simulink model "SignosPatologia"  (R2020a)
settings: Solver=FixedStepAuto  StartTime=0.0  StopTime=10.0  RelTol=1e-3
undefined symbols (not defined in the file): A1, alphaCo2, c1, c2, c3, Ca, Ce, Ci, Cv, d, Ed, epsilon, Es0, gananciaOut, K, offsetMaxFinder, omega0, Pex, picoR, Pset, Ra, Re0, Ri, Rlv, Rv, T, tau, tau1, tau2, Tdia, Ve0
libraries: androiduilib x6, simulink x4, dspswit3 x2
settings Model: Creator=luisi  LastModifiedBy=luisi
settings OptimizationCC: EnhancedBackFolding=on  PassReuseOutputArgsAs=Individual arguments  ZeroExternalMemoryAtStartup=off  ZeroInternalMemoryAtStartup=off  MaxStackSize=64  OptimizeBlockOrder=speed  DifferentSizesBufferReuse=on  OptimizationCustomize=off  EfficientTunableParamExpr=on
settings DebuggingCC: ParameterTunabilityLossMsg=error
settings HardwareCC: ProdBitPerPointer=32  ProdBitPerSizeT=32  ProdBitPerPtrDiffT=32  ProdLargestAtomicInteger=Long  ProdLargestAtomicFloat=Double  ProdWordSize=32  ProdHWDeviceType=ARM Compatible->ARM Cortex
settings SFSimCC: MATLABDynamicMemAlloc=off
settings RTWCC: SystemTargetFile=ert.tlc  HardwareBoard=Android Device  TemplateMakefile=ert_default_tmf  RTWVerbose=off  Toolchain=Android SDK/NDK Tools
settings CodeAppCC: ForceParamTrailComments=on  IgnoreCustomStorageClasses=off  OperatorAnnotations=on  SimulinkDataObjDesc=on  SFDataObjDesc=on  InsertBlockDesc=on
settings ERTTargetCC: SupportContinuousTime=on

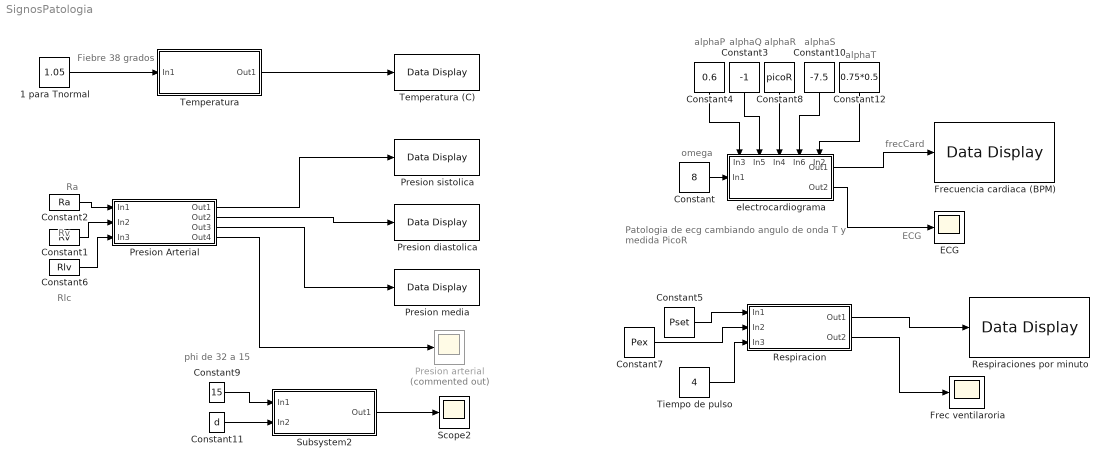
== system SignosPatologia ==
  note: Ra
  note: phi de 32 a 15
  note: Patologia de ecg cambiando angulo de onda T
      |  y medida PicoR
  note: Fiebre 38 grados
  note: alphaR
  note: ECG
  note: alphaQ
  note: alphaP
  note: alphaT
  note: alphaS
  note: omega
  note: frecCard
  note: Rv
  note: Rlc
  1 para Tnormal : Constant  Value=1.05
  Constant : Constant  Value=8
  Constant1 : Constant  Value=Rv
  Constant10 : Constant  Value=-7.5
  Constant11 : Constant  Value=d
  Constant12 : Constant  Value=0.75*0.5
  Constant2 : Constant  Value=Ra
  Constant3 : Constant  Value=-1
  Constant4 : Constant  Value=0.6
  Constant5 : Constant  Value=Pset
  Constant6 : Constant  Value=Rlv
  Constant7 : Constant  Value=Pex
  Constant8 : Constant  Value=picoR
  Constant9 : Constant  Value=15
  ECG : Scope
      settings: AttributesFormatString=%<AxesScaling>
  Frec ventilaroria : Scope
  Frecuencia cardiaca (BPM) : androiduilib/Data Display  DataDisplayId=SignosPatologia/Frecuencia_cardiaca_(BPM)  Format=Float  Precision=6  SimulateUsing=Code generation  blockPlatform=Android
      settings: SourceProductBaseCode=ANDROID
  Presion Arterial : Subsystem
  Presion arterial : Scope  Commented=on
  Presion diastolica : androiduilib/Data Display  DataDisplayId=SignosPatologia/Presion_diastolica  Format=Float  Precision=6  SimulateUsing=Code generation  blockPlatform=Android
      settings: SourceProductBaseCode=ANDROID
  Presion media : androiduilib/Data Display  DataDisplayId=SignosPatologia/Presion_media  Format=Float  Precision=6  SimulateUsing=Code generation  blockPlatform=Android
      settings: SourceProductBaseCode=ANDROID
  Presion sistolica : androiduilib/Data Display  DataDisplayId=SignosPatologia/Presion_sistolica  Format=Float  Precision=6  SimulateUsing=Code generation  blockPlatform=Android
      settings: SourceProductBaseCode=ANDROID
  Respiracion : Subsystem
  Respiraciones por minuto : androiduilib/Data Display  DataDisplayId=SignosPatologia/Respiraciones_por_minuto  Format=Float  Precision=6  SimulateUsing=Code generation  blockPlatform=Android
      settings: SourceProductBaseCode=ANDROID
  Scope2 : Scope
  Subsystem2 : Subsystem
  Temperatura : Subsystem
  Temperatura (C) : androiduilib/Data Display  DataDisplayId=SignosPatologia/Temperatura_(C)  Format=Float  Precision=6  SimulateUsing=Code generation  blockPlatform=Android
      settings: SourceProductBaseCode=ANDROID
  Tiempo de pulso : Constant  Value=4
  electrocardiograma : Subsystem
      settings: PortSchema="{\"entries\":[{\"content\":{\"sides\":[{\"content\":{\"connectorIds\":[\"In1\"]},\"type\":\"ConnectorPlacement.EquallySpacedRectSide\",\"uuid\":\"28011a65-da2e-41a8-8a5a-207c074f97f9\"},{\"content\":{\"connectorIds\":[\"Out1\",\"Out2\"],\"side\":\"RIGHT\"},\"type\":\"ConnectorPlacement.EquallySpacedRectSide\",\"uuid\":\"adec610a-f47f-48bc-af05-027a0272bce0\"},{\"content\":{\"connectorIds\":[\"In2\",\"In3\",\"In4\",\"In5\",\"In6\"],\"side\":\"TOP\"},\"type\":\"ConnectorPlacement.EquallySpacedRectSide\",\"uuid\":\"45565275-fa9c-45e2-aeb7-03b042b7619a\"}]},\"type\":\"ConnectorPlacement.EquallySpacedConnector\",\"uuid\":\"6408496b-6851-4df8-8646-e1f498398f76\"}],\"packageUris\":[\"http://schema.mathworks.com/mf0/Connector/19700101\"],\"version\":\"1.0\"}"
  wires:
  Temperatura/1(Out1) -> Temperatura (C)/1
  1 para Tnormal/1 -> Temperatura/1(In1)
  Presion Arterial/2(Out2) -> Presion diastolica/1
  Presion Arterial/3(Out3) -> Presion media/1
  Constant2/1 -> Presion Arterial/1(In1)
  Constant6/1 -> Presion Arterial/3(In3)
  Presion Arterial/1(Out1) -> Presion sistolica/1
  Constant1/1 -> Presion Arterial/2(In2)
  Constant8/1 -> electrocardiograma/4(In4)
  Constant/1 -> electrocardiograma/1(In1)
  electrocardiograma/1(Out1) -> Frecuencia cardiaca (BPM)/1
  electrocardiograma/2(Out2) -> ECG/1
  Constant4/1 -> electrocardiograma/2(In3)
  Constant12/1 -> electrocardiograma/6(In2)
  Constant10/1 -> electrocardiograma/5(In6)
  Constant3/1 -> electrocardiograma/3(In5)
  Presion Arterial/4(Out4) -> Presion arterial/1
  Constant7/1 -> Respiracion/2(In2)
  Constant5/1 -> Respiracion/1(In1)
  Respiracion/1(Out1) -> Respiraciones por minuto/1
  Respiracion/2(Out2) -> Frec ventilaroria/1
  Tiempo de pulso/1 -> Respiracion/3(In3)
  Constant9/1 -> Subsystem2/1(In1)
  Subsystem2/1(Out1) -> Scope2/1
  Constant11/1 -> Subsystem2/2(In2)

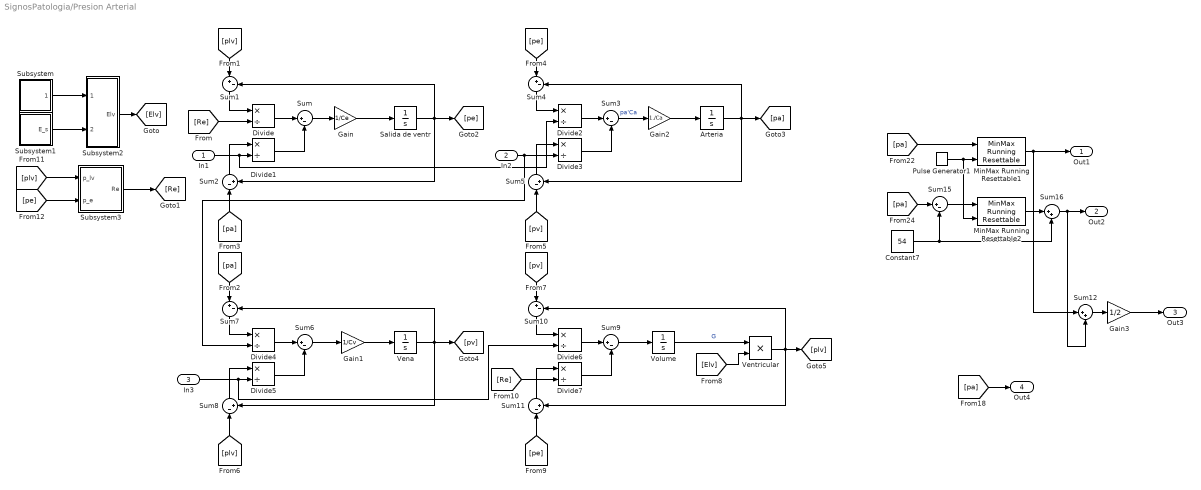
== system SignosPatologia/Presion Arterial ==
  In1 : Inport
  In2 : Inport  Port=2
  In3 : Inport  Port=3
  Arteria : Integrator  InitialCondition=70
  Constant7 : Constant  Value=54
  Divide{,1..7} (8 alike) : Product  Inputs=*/
  Gain : Gain  Gain=1/Ce
  Gain1 : Gain  Gain=1/Cv
  Gain2 : Gain  Gain=1./Ca
  Gain3 : Gain  Gain=1/2
  MinMax Running Resettable1 : simulink/Math Operations/MinMax Running Resettable  Function=max  vinit=70
  MinMax Running Resettable2 : simulink/Math Operations/MinMax Running Resettable  Function=min  vinit=0.0
  Pulse Generator1 : DiscretePulseGenerator  PulseType=Time based  Period=8  PulseWidth=5
  Salida de ventr : Integrator  InitialCondition=49.896
  Subsystem : Subsystem
  Subsystem1 : Subsystem
  Subsystem2 : Subsystem
  Subsystem3 : Subsystem
  Sum{,1,3..4,6..7,9..10,15} (9 alike) : Sum  Inputs=|+-
  Sum{2,5,8,11} (4 alike) : Sum  Inputs=|-+
  Sum12 : Sum  Inputs=|++
  Sum16 : Sum  Inputs=|++
  Vena : Integrator  InitialCondition=16.628
  Ventricular : Product
  Volume : Integrator  InitialCondition=49.714/0.0655
  Out1 : Outport
  Out2 : Outport  Port=2
  Out3 : Outport  Port=3
  Out4 : Outport  Port=4
  wires:
  Sum12/1 -> Gain3/1
  Gain3/1 -> Out3/1
  Sum16/1 -> Sum12/2, Out2/1
  MinMax Running Resettable2/1 -> Sum16/1
  Sum3/1 -> Gain2/1  "pa'Ca"
  [pa] -> MinMax Running Resettable1/1
  Sum10/1 -> Divide6/1
  MinMax Running Resettable1/1 -> Sum12/1, Out1/1
  Subsystem2/1(Elv) -> [Elv]
  Constant7/1 -> Sum16/2, Sum15/2
  Salida de ventr/1 -> [pe], Sum2/2, Sum1/2
  [pa] -> Sum15/1
  Divide6/1 -> Sum9/1
  Pulse Generator1/1 -> MinMax Running Resettable2/2, MinMax Running Resettable1/2
  [Elv] -> Ventricular/2
  [pa] -> Out4/1
  Gain/1 -> Salida de ventr/1
  [Re] -> Divide/2
  In2/1 -> Divide4/2, Divide3/2
  Sum5/1 -> Divide3/1
  [plv] -> Subsystem3/1(p_lv)
  Divide/1 -> Sum/1
  [plv] -> Sum1/1
  [pv] -> Sum10/1
  Ventricular/1 -> Sum10/2, [plv], Sum11/2
  Sum15/1 -> MinMax Running Resettable2/1
  [pe] -> Sum4/1
  [pe] -> Subsystem3/2(p_e)
  Sum9/1 -> Volume/1
  [plv] -> Sum8/1
  Gain1/1 -> Vena/1
  [pv] -> Sum5/1
  Divide7/1 -> Sum9/2
  In3/1 -> Divide6/2, Divide5/2
  Gain2/1 -> Arteria/1
  Sum8/1 -> Divide5/1
  Sum11/1 -> Divide7/1
  Divide2/1 -> Sum3/1
  [pe] -> Sum11/1
  [pa] -> Sum7/1
  Sum7/1 -> Divide4/1
  Vena/1 -> [pv], Sum8/2, Sum7/2
  Divide3/1 -> Sum3/2
  Sum6/1 -> Gain1/1
  Volume/1 -> Ventricular/1  "G"
  Divide5/1 -> Sum6/2
  Divide4/1 -> Sum6/1
  Arteria/1 -> Sum5/2, Sum4/2, [pa]
  [pa] -> Sum2/1
  [Re] -> Divide7/2
  Sum2/1 -> Divide1/1
  Sum1/1 -> Divide/1
  Sum/1 -> Gain/1
  Sum4/1 -> Divide2/1
  Subsystem3/1(Re) -> [Re]
  Subsystem/1(alpha_t) -> Subsystem2/1(alpha)
  Subsystem1/1(E_s) -> Subsystem2/2(E_s)
  Divide1/1 -> Sum/2
  In1/1 -> Divide2/2, Divide1/2

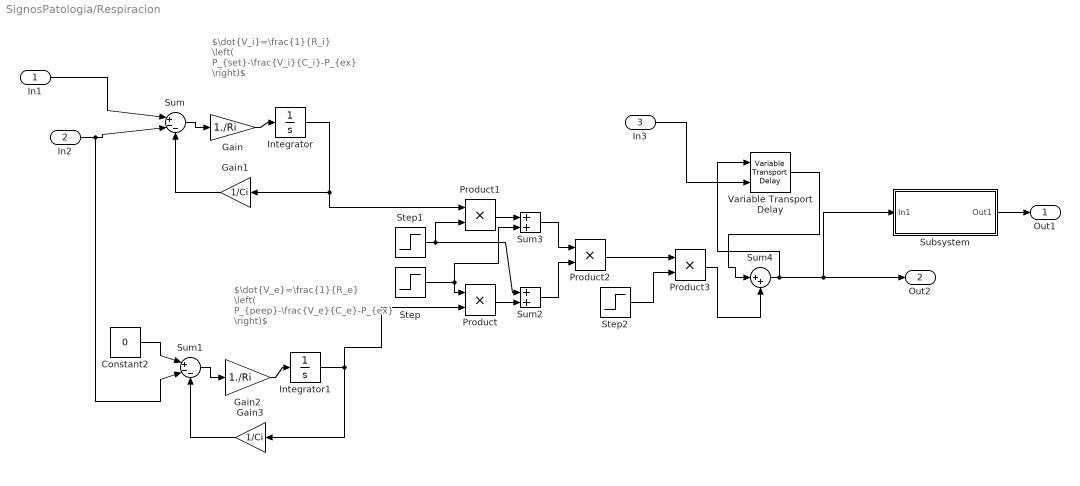
== system SignosPatologia/Respiracion ==
  note: $\dot{V_i}=\frac{1}{R_i} \left( P_{set}-\frac{V_i}{C_i}-P_{ex} \right)$
  note: $\dot{V_e}=\frac{1}{R_e} \left( P_{peep}-\frac{V_e}{C_e}-P_{ex} \right)$
  In1 : Inport
  In2 : Inport  Port=2
  In3 : Inport  Port=3
  Constant2 : Constant  Value=0
  Gain : Gain  Gain=1./Ri
  Gain1 : Gain  Gain=1/Ci
  Gain2 : Gain  Gain=1./Ri
  Gain3 : Gain  Gain=1/Ci
  Integrator : Integrator
  Integrator1 : Integrator  InitialCondition=Ve0
  Product{,1..3} (4 alike) : Product
  Step : Step  Time=2  SampleTime=0
  Step1 : Step  Time=2  Before=1  After=0  SampleTime=0
  Step2 : Step  Time=4  Before=1  After=0  SampleTime=0
  Subsystem : Subsystem
  Sum : Sum  Inputs=|+--
  Sum1 : Sum  Inputs=|+--
  Sum2 : Sum
  Sum3 : Sum
  Sum4 : Sum  Inputs=|++
  Variable Transport Delay : VariableTransportDelay  VariableDelayType=Variable transport delay  MaximumDelay=10
  Out1 : Outport
  Out2 : Outport  Port=2
  wires:
  Sum3/1 -> Product2/1
  Sum2/1 -> Product2/2
  Gain3/1 -> Sum1/3
  Integrator1/1 -> Product/2, Gain3/1
  Product2/1 -> Product3/1
  Product1/1 -> Sum3/1
  Step2/1 -> Product3/2
  Product3/1 -> Sum4/2
  Integrator/1 -> Product1/1, Gain1/1
  Step/1 -> Product/1, Sum3/2
  Product/1 -> Sum2/2
  Sum4/1 -> Variable Transport Delay/1, Out2/1, Subsystem/1(In1)
  Gain2/1 -> Integrator1/1
  Variable Transport Delay/1 -> Sum4/1
  Gain1/1 -> Sum/3
  Subsystem/1(Out1) -> Out1/1
  Sum1/1 -> Gain2/1
  Step1/1 -> Sum2/1, Product1/2
  In2/1 -> Sum1/2, Sum/2
  Constant2/1 -> Sum1/1
  Gain/1 -> Integrator/1
  Sum/1 -> Gain/1
  In1/1 -> Sum/1
  In3/1 -> Variable Transport Delay/2

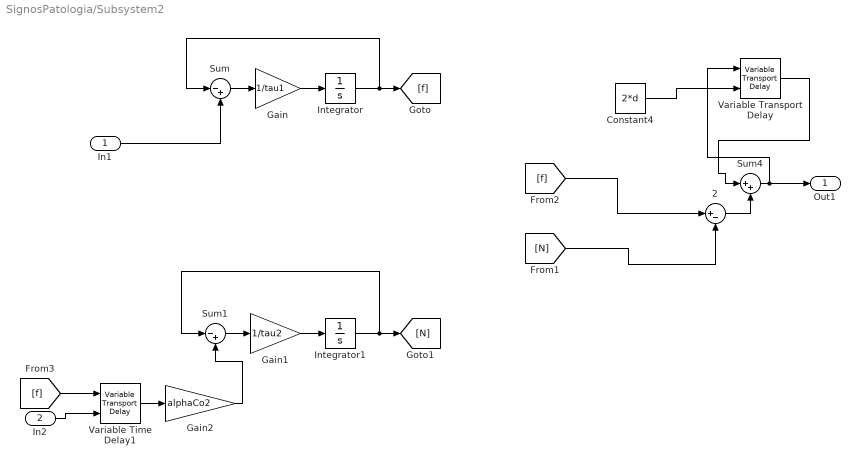
== system SignosPatologia/Subsystem2 ==
  In1 : Inport
  In2 : Inport  Port=2
  2 : Sum  Inputs=|+-
  Constant4 : Constant  Value=2*d
  Gain : Gain  Gain=1/tau1
  Gain1 : Gain  Gain=1/tau2
  Gain2 : Gain  Gain=alphaCo2
  Integrator : Integrator
  Integrator1 : Integrator
  Sum : Sum  Inputs=|-+
  Sum1 : Sum  Inputs=|-+
  Sum4 : Sum  Inputs=|++
  Variable Time Delay1 : VariableTransportDelay  MaximumDelay=10
  Variable Transport Delay : VariableTransportDelay  VariableDelayType=Variable transport delay  MaximumDelay=10
  Out1 : Outport
  wires:
  In1/1 -> Sum/2
  Sum1/1 -> Gain1/1
  Gain1/1 -> Integrator1/1
  Integrator1/1 -> [N], Sum1/1
  Sum4/1 -> Out1/1, Variable Transport Delay/1
  Integrator/1 -> [f], Sum/1
  Gain/1 -> Integrator/1
  Constant4/1 -> Variable Transport Delay/2
  [f] -> 2/1
  [N] -> 2/2
  [f] -> Variable Time Delay1/1
  Gain2/1 -> Sum1/2
  Sum/1 -> Gain/1
  Variable Transport Delay/1 -> Sum4/1
  In2/1 -> Variable Time Delay1/2
  2/1 -> Sum4/2
  Variable Time Delay1/1 -> Gain2/1

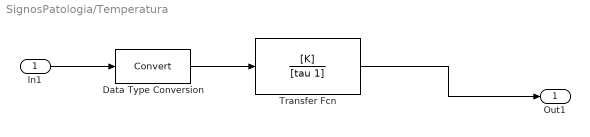
== system SignosPatologia/Temperatura ==
  In1 : Inport
  Data Type Conversion : DataTypeConversion
  Transfer Fcn : TransferFcn  Numerator=[K]  Denominator=[tau 1]
  Out1 : Outport
  wires:
  Data Type Conversion/1 -> Transfer Fcn/1
  Transfer Fcn/1 -> Out1/1
  In1/1 -> Data Type Conversion/1

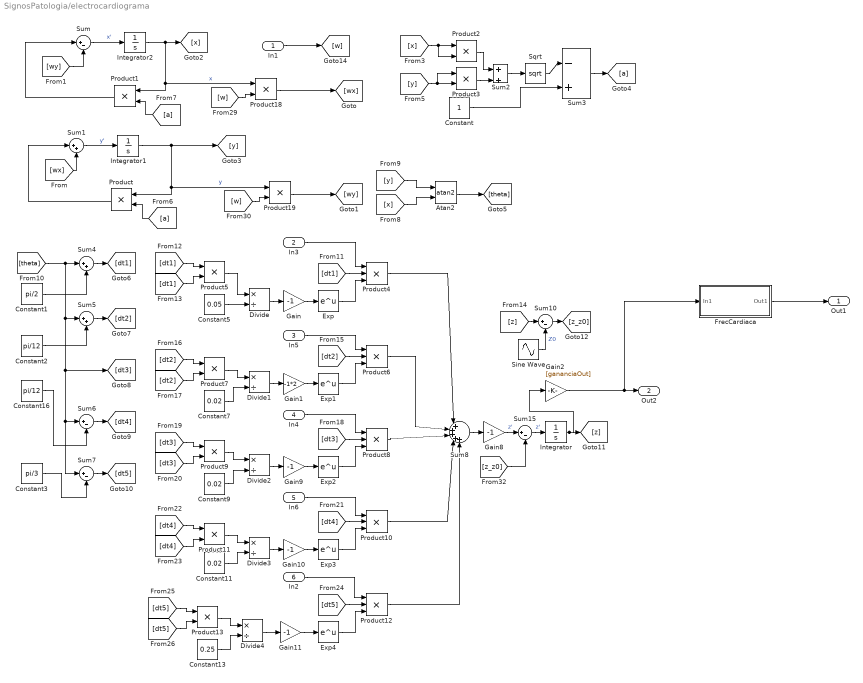
== system SignosPatologia/electrocardiograma ==
  In1 : Inport
  In3 : Inport  Port=2
  In5 : Inport  Port=3
  In4 : Inport  Port=4
  In6 : Inport  Port=5
  In2 : Inport  Port=6
  Atan2 : Trigonometry  Operator=atan2
  Constant : Constant
  Constant1 : Constant  Value=pi/2
  Constant11 : Constant  Value=0.02
  Constant13 : Constant  Value=0.25
  Constant16 : Constant  Value=pi/12
  Constant2 : Constant  Value=pi/12
  Constant3 : Constant  Value=pi/3
  Constant5 : Constant  Value=0.05
  Constant7 : Constant  Value=0.02
  Constant9 : Constant  Value=0.02
  Divide{,1..4} (5 alike) : Product  Inputs=*/
  Exp{,1..4} (5 alike) : Math  SaturateOnIntegerOverflow=on
  FrecCardiaca : Subsystem
  Gain{,8..11} (5 alike) : Gain  Gain=-1
  Gain1 : Gain  Gain=-1*2
  Gain2 : Gain  Gain=[gananciaOut]
  Integrator : Integrator  InitialCondition=1000
  Integrator1 : Integrator
  Integrator2 : Integrator  InitialCondition=2
  Product{,1..3,5,7,9,11,13,18..19} (11 alike) : Product
  Product{4,6,8,10,12} (5 alike) : Product  Inputs=3
  Sine Wave : Sin  Amplitude=0.15e-3  Frequency=0.25  SampleTime=0
  Sqrt : Sqrt  SaturateOnIntegerOverflow=on
  Sum{,6..7,10,15} (5 alike) : Sum  Inputs=|+-
  Sum{1..2,4..5} (4 alike) : Sum  Inputs=|++
  Sum3 : Sum  Inputs=|-+
  Sum8 : Sum  Inputs=|+++++
  Out1 : Outport
  Out2 : Outport  Port=2
  wires:
  [dt2] -> Product6/2
  Product4/1 -> Sum8/1
  [x] -> Atan2/2
  Product3/1 -> Sum2/2
  [y] -> Atan2/1
  FrecCardiaca/1(Out1) -> Out1/1
  Product/1 -> Sum1/1
  Product5/1 -> Divide/1
  [dt2] -> Product7/2
  Gain/1 -> Exp/1
  Product1/1 -> Sum/1
  Constant/1 -> Sum3/2
  Divide1/1 -> Gain1/1
  Exp4/1 -> Product12/3
  Exp3/1 -> Product10/3
  Gain11/1 -> Exp4/1
  Exp/1 -> Product4/3
  In2/1 -> Product12/1
  Constant11/1 -> Divide3/2
  Divide2/1 -> Gain9/1
  [dt1] -> Product4/2
  Product18/1 -> [wx]
  Sum2/1 -> Sqrt/1
  [a] -> Product1/2
  Constant1/1 -> Sum4/2
  Product8/1 -> Sum8/3
  Exp2/1 -> Product8/3
  Product11/1 -> Divide3/1
  [dt3] -> Product9/2
  Integrator1/1 -> [y], Product19/1, Product/1  "y"
  Constant5/1 -> Divide/2
  Product7/1 -> Divide1/1
  [dt4] -> Product11/1
  Sqrt/1 -> Sum3/1
  Product13/1 -> Divide4/1
  Gain10/1 -> Exp3/1
  In4/1 -> Product8/1
  [dt1] -> Product5/1
  Gain1/1 -> Exp1/1
  [dt5] -> Product13/2
  [dt4] -> Product11/2
  [dt1] -> Product5/2
  Constant9/1 -> Divide2/2
  [dt5] -> Product12/2
  Divide/1 -> Gain/1
  Divide4/1 -> Gain11/1
  [dt5] -> Product13/1
  Product12/1 -> Sum8/5
  Product6/1 -> Sum8/2
  Constant13/1 -> Divide4/2
  Product10/1 -> Sum8/4
  Sum5/1 -> [dt2]
  [dt4] -> Product10/2
  Sine Wave/1 -> Sum10/2  "Z0"
  Sum6/1 -> [dt4]
  Sum1/1 -> Integrator1/1  "y'"
  [dt3] -> Product9/1
  Atan2/1 -> [theta]
  [w] -> Product19/2
  Sum7/1 -> [dt5]
  In5/1 -> Product6/1
  Sum10/1 -> [z_z0]
  Gain8/1 -> Sum15/1  "z'"
  Integrator/1 -> Gain2/1, [z]
  [dt3] -> Product8/2
  [theta] -> Sum7/1, Sum6/1, [dt3], Sum5/1, Sum4/1
  [z_z0] -> Sum15/2
  [a] -> Product/2
  Integrator2/1 -> [x], Product1/1, Product18/1  "x"
  Exp1/1 -> Product6/3
  Constant16/1 -> Sum6/2
  Sum4/1 -> [dt1]
  In3/1 -> Product4/1
  Sum15/1 -> Integrator/1  "z'"
  Product19/1 -> [wy]
  Sum/1 -> Integrator2/1  "x'"
  [wx] -> Sum1/2
  Constant3/1 -> Sum7/2
  [y] -> Product3/1, Product3/2
  [wy] -> Sum/2
  Constant2/1 -> Sum5/2
  Product9/1 -> Divide2/1
  Constant7/1 -> Divide1/2
  Sum3/1 -> [a]
  [x] -> Product2/2, Product2/1
  [dt2] -> Product7/1
  [z] -> Sum10/1
  Gain9/1 -> Exp2/1
  [w] -> Product18/2
  Product2/1 -> Sum2/1
  Gain2/1 -> Out2/1, FrecCardiaca/1(In1)
  Divide3/1 -> Gain10/1
  Sum8/1 -> Gain8/1
  In1/1 -> [w]
  In6/1 -> Product10/1

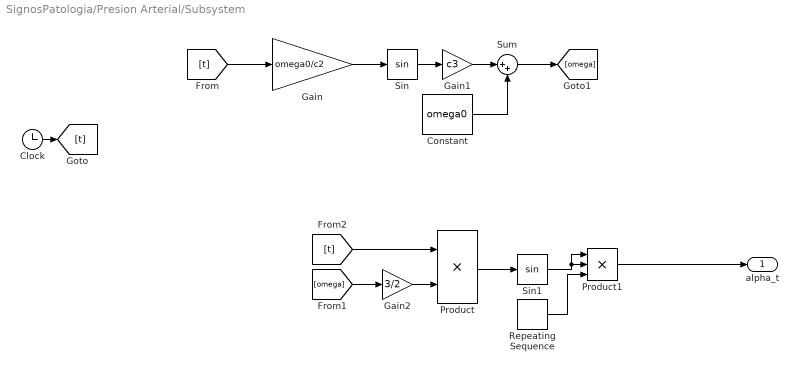
== system SignosPatologia/Presion Arterial/Subsystem ==
  Clock : Clock
  Constant : Constant  Value=omega0
  Gain : Gain  Gain=omega0/c2
  Gain1 : Gain  Gain=c3
  Gain2 : Gain  Gain=3/2
  Product : Product
  Product1 : Product  Inputs=3
  Repeating Sequence : simulink/Sources/Repeating Sequence  rep_seq_t=[0 Tdia Tdia+0.001 T]  rep_seq_y=[0 0 1 1]
  Sin : Trigonometry
  Sin1 : Trigonometry
  Sum : Sum  Inputs=|++
  alpha_t : Outport
  wires:
  Clock/1 -> [t]
  [t] -> Gain/1
  Gain/1 -> Sin/1
  Sin/1 -> Gain1/1
  Gain1/1 -> Sum/1
  Constant/1 -> Sum/2
  Sum/1 -> [omega]
  [t] -> Product/1
  [omega] -> Gain2/1
  Product/1 -> Sin1/1
  Sin1/1 -> Product1/1, Product1/2
  Product1/1 -> alpha_t/1
  Gain2/1 -> Product/2
  Repeating Sequence/1 -> Product1/3

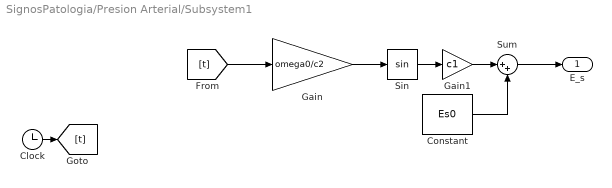
== system SignosPatologia/Presion Arterial/Subsystem1 ==
  Clock : Clock
  Constant : Constant  Value=Es0
  Gain : Gain  Gain=omega0/c2
  Gain1 : Gain  Gain=c1
  Sin : Trigonometry
  Sum : Sum  Inputs=|++
  E_s : Outport
  wires:
  Sum/1 -> E_s/1
  Constant/1 -> Sum/2
  Gain1/1 -> Sum/1
  Sin/1 -> Gain1/1
  Gain/1 -> Sin/1
  [t] -> Gain/1
  Clock/1 -> [t]

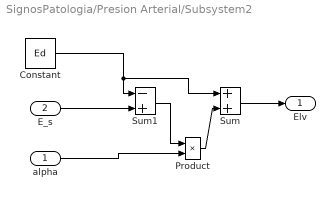
== system SignosPatologia/Presion Arterial/Subsystem2 ==
  alpha : Inport
  E_s : Inport  Port=2
  Constant : Constant  Value=Ed
  Product : Product
  Sum : Sum
  Sum1 : Sum  Inputs=-+
  Elv : Outport
  wires:
  Constant/1 -> Sum1/1, Sum/1
  E_s/1 -> Sum1/2
  alpha/1 -> Product/2
  Sum1/1 -> Product/1
  Product/1 -> Sum/2
  Sum/1 -> Elv/1

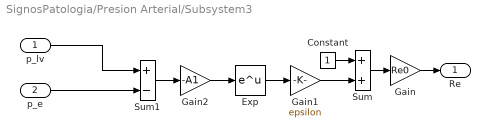
== system SignosPatologia/Presion Arterial/Subsystem3 ==
  p_lv : Inport
  p_e : Inport  Port=2
  Constant : Constant
  Exp : Math  SaturateOnIntegerOverflow=on
  Gain : Gain  Gain=Re0
  Gain1 : Gain  Gain=epsilon
  Gain2 : Gain  Gain=-A1
  Sum : Sum
  Sum1 : Sum  Inputs=+-
  Re : Outport
  wires:
  Sum/1 -> Gain/1
  Gain/1 -> Re/1
  Constant/1 -> Sum/1
  Gain1/1 -> Sum/2
  Exp/1 -> Gain1/1
  p_lv/1 -> Sum1/1
  p_e/1 -> Sum1/2
  Gain2/1 -> Exp/1
  Sum1/1 -> Gain2/1

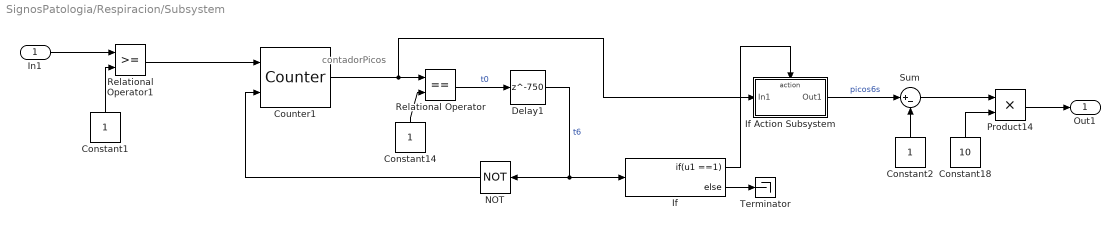
== system SignosPatologia/Respiracion/Subsystem ==
  note: contadorPicos
  In1 : Inport
  Constant1 : Constant
  Constant14 : Constant
  Constant18 : Constant  Value=10
  Constant2 : Constant
  Counter1 : dspswit3/Counter  Direction=Up  CountEvent=Rising edge  CounterSize=User defined  MaxCount=100  InitialCount=0  Output=Count  HitValue=32  ResetInput=on  SamplesPerFrame=1  Ts=1  CntDtype=double  HitDtype=Logical
  Delay1 : Delay  DelayLength=750  SampleTime=0.008
  If : If  IfExpression=u1 ==1
  If Action Subsystem : Subsystem  TreatAsAtomicUnit=on
  NOT : Logic  Operator=NOT  IconShape=distinctive  AllPortsSameDT=off  OutDataTypeStr=boolean
  Product14 : Product
  Relational Operator : RelationalOperator  Operator===  OutDataTypeStr=boolean  RndMeth=Simplest
  Relational Operator1 : RelationalOperator  OutDataTypeStr=boolean  RndMeth=Simplest
  Sum : Sum  Inputs=|+-
  Terminator : Terminator
  Out1 : Outport
  wires:
  Relational Operator1/1 -> Counter1/1
  Relational Operator/1 -> Delay1/1  "t0"
  Product14/1 -> Out1/1
  If/2 -> Terminator/1
  Constant18/1 -> Product14/2
  Delay1/1 -> NOT/1, If/1  "t6"
  NOT/1 -> Counter1/2
  In1/1 -> Relational Operator1/1
  Counter1/1 -> If Action Subsystem/1(In1), Relational Operator/1
  If/1 -> If Action Subsystem/Action
  Constant14/1 -> Relational Operator/2
  Constant1/1 -> Relational Operator1/2
  If Action Subsystem/1(Out1) -> Sum/1  "picos6s"
  Sum/1 -> Product14/1
  Constant2/1 -> Sum/2

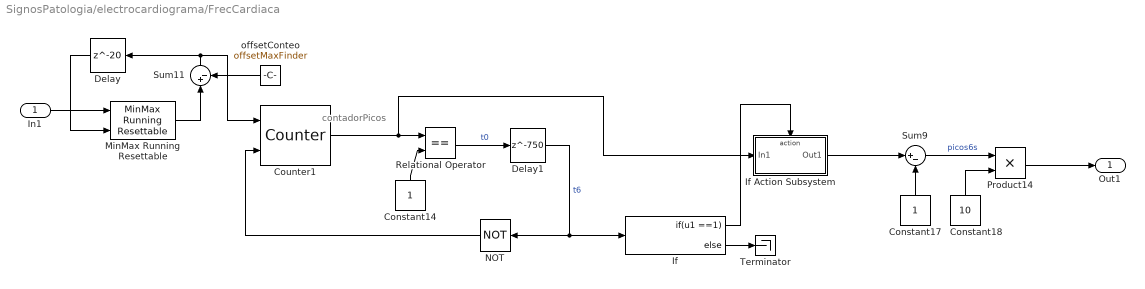
== system SignosPatologia/electrocardiograma/FrecCardiaca ==
  note: contadorPicos
  In1 : Inport
  Constant14 : Constant
  Constant17 : Constant
  Constant18 : Constant  Value=10
  Counter1 : dspswit3/Counter  Direction=Up  CountEvent=Rising edge  CounterSize=User defined  MaxCount=100  InitialCount=0  Output=Count  HitValue=32  ResetInput=on  SamplesPerFrame=1  Ts=1  CntDtype=double  HitDtype=Logical
  Delay : Delay  DelayLength=20  InitialCondition=[offsetMaxFinder]  SampleTime=0.008
  Delay1 : Delay  DelayLength=750  SampleTime=0.008
  If : If  IfExpression=u1 ==1
  If Action Subsystem : Subsystem  TreatAsAtomicUnit=on
  MinMax Running Resettable : simulink/Math Operations/MinMax Running Resettable  Function=max  vinit=offsetMaxFinder
  NOT : Logic  Operator=NOT  IconShape=distinctive  AllPortsSameDT=off  OutDataTypeStr=boolean
  Product14 : Product
  Relational Operator : RelationalOperator  Operator===  OutDataTypeStr=boolean  RndMeth=Simplest
  Sum11 : Sum  Inputs=|+-
  Sum9 : Sum  Inputs=|+-
  Terminator : Terminator
  offsetConteo : Constant  Value=offsetMaxFinder
  Out1 : Outport
  wires:
  NOT/1 -> Counter1/2
  Sum9/1 -> Product14/1  "picos6s"
  If/2 -> Terminator/1
  Product14/1 -> Out1/1
  If Action Subsystem/1(Out1) -> Sum9/1
  If/1 -> If Action Subsystem/Action
  Delay1/1 -> NOT/1, If/1  "t6"
  Constant17/1 -> Sum9/2
  Relational Operator/1 -> Delay1/1  "t0"
  Constant14/1 -> Relational Operator/2
  In1/1 -> MinMax Running Resettable/1
  Counter1/1 -> If Action Subsystem/1(In1), Relational Operator/1
  MinMax Running Resettable/1 -> Sum11/1
  offsetConteo/1 -> Sum11/2
  Constant18/1 -> Product14/2
  Delay/1 -> MinMax Running Resettable/2
  Sum11/1 -> Counter1/1, Delay/1

== system SignosPatologia/Respiracion/Subsystem/If Action Subsystem ==
  In1 : Inport
  Action Port : ActionPort  ActionPortLabel=if(u1 ==1)
  Out1 : Outport
  wires:
  In1/1 -> Out1/1

== system SignosPatologia/electrocardiograma/FrecCardiaca/If Action Subsystem ==
  In1 : Inport
  Action Port : ActionPort  ActionPortLabel=if(u1 ==1)
  Out1 : Outport
  wires:
  In1/1 -> Out1/1
